simulink model "coord_trans_block_example_model"  (R2025b)
settings: Solver=VariableStepAuto  StartTime=0.0  StopTime=10.0  RelTol=1e-3
undefined symbols (not defined in the file): Angle, Axis
libraries: robotcorelib x3
settings Model: Creator=The MathWorks, Inc.  LastModifiedBy=The MathWorks, Inc.
settings SolverCC: AlgebraicLoopSolver=TrustRegion
settings DataIOCC: ReturnWorkspaceOutputs=off
settings DebuggingCC: UnconnectedInputMsg=warning  UnconnectedOutputMsg=warning  UnconnectedLineMsg=warning  ArithmeticOperatorsInVariantConditions=warning
settings ModelReferenceCC: EnableRefExpFcnMdlSchedulingChecks=on
settings SFSimCC: SimUseLocalCustomCode=off  CustomCodeUndefinedFunction=UseInterfaceOnly
settings RTWCC: RTWUseLocalCustomCode=off  GPUComputeCapability=3.5

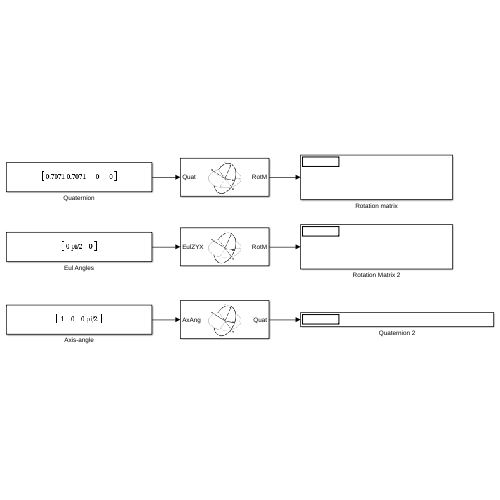
[thumbnail: Simulink's stored preview of the top-level diagram]
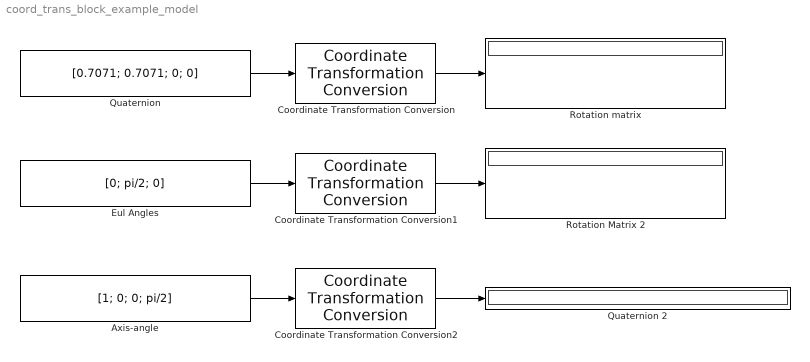
== system coord_trans_block_example_model ==
  Axis-angle : Constant  Value=[1; 0; 0; pi/2]
  Coordinate Transformation Conversion : robotcorelib/Coordinate Transformation Conversion  InputRepresentation=Quaternion  InputEulerSequence=ZYX  ShowTrVecInputPort=on  OutputRepresentation=Rotation Matrix  OutputEulerSequence=ZYX  ShowTrVecOutputPort=on  SimulateUsing=Interpreted execution
  Coordinate Transformation Conversion1 : robotcorelib/Coordinate Transformation Conversion  InputRepresentation=Euler Angles  InputEulerSequence=ZYX  ShowTrVecInputPort=on  OutputRepresentation=Rotation Matrix  OutputEulerSequence=ZYX  ShowTrVecOutputPort=on  SimulateUsing=Interpreted execution
  Coordinate Transformation Conversion2 : robotcorelib/Coordinate Transformation Conversion  InputRepresentation=Axis-Angle  InputEulerSequence=ZYX  ShowTrVecInputPort=on  OutputRepresentation=Quaternion  OutputEulerSequence=ZYX  ShowTrVecOutputPort=on  SimulateUsing=Interpreted execution
  Eul Angles : Constant  Value=[0; pi/2; 0]
  Quaternion : Constant  Value=[0.7071; 0.7071; 0; 0]
  Quaternion 2 : Display
  Rotation Matrix 2 : Display
  Rotation matrix : Display
  wires:
  Quaternion/1 -> Coordinate Transformation Conversion/1
  Coordinate Transformation Conversion/1 -> Rotation matrix/1
  Eul Angles/1 -> Coordinate Transformation Conversion1/1
  Coordinate Transformation Conversion1/1 -> Rotation Matrix 2/1
  Axis-angle/1 -> Coordinate Transformation Conversion2/1
  Coordinate Transformation Conversion2/1 -> Quaternion 2/1
